simulink model "MBD2_problem3"  (R2020b)
settings: Solver=VariableStepAuto  StartTime=0.0  StopTime=100  RelTol=1e-3
InitFcn:
  | M = 1000;
  | b = 50;
  | u = 500;
  | Kp=1750;
  | Ki=800;
  | Ts=0.01;
settings Model: Creator=Lenovo  LastModifiedBy=Lenovo

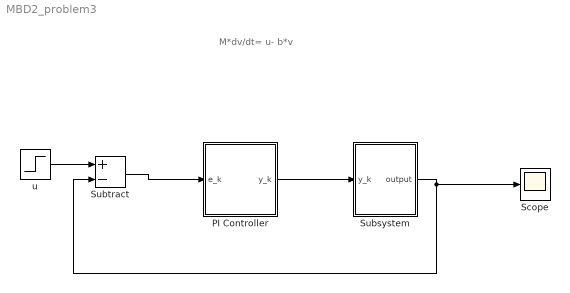
== system MBD2_problem3 ==
  note: M*dv/dt= u- b*v
  PI Controller : Subsystem
  Scope : Scope
  Subsystem : Subsystem
  Subtract : Sum  Inputs=+-
  u : Step  Time=0  SampleTime=0
  wires:
  Subsystem/1(output) -> Subtract/2, Scope/1
  u/1 -> Subtract/1
  Subtract/1 -> PI Controller/1(e_k)
  PI Controller/1(y_k) -> Subsystem/1(y_k)

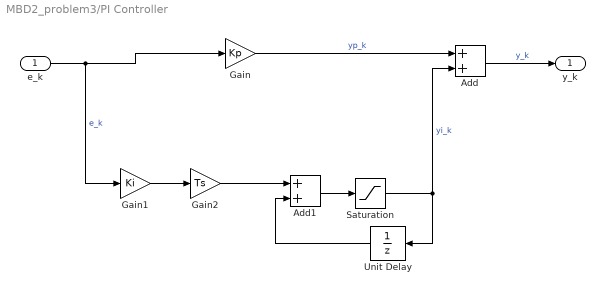
== system MBD2_problem3/PI Controller ==
  e_k : Inport  OutDataTypeStr=double  PortDimensions=1  SampleTime=0
  Add : Sum
  Add1 : Sum
  Gain : Gain  Gain=Kp
  Gain1 : Gain  Gain=Ki
  Gain2 : Gain  Gain=Ts
  Saturation : Saturate  UpperLimit=1  LowerLimit=-1
  Unit Delay : UnitDelay  SampleTime=-1  HasFrameUpgradeWarning=on
  y_k : Outport  OutDataTypeStr=double  PortDimensions=1  SampleTime=0
  wires:
  Gain2/1 -> Add1/1
  Add1/1 -> Saturation/1
  e_k/1 -> Gain/1, Gain1/1  "e_k"
  Gain1/1 -> Gain2/1
  Add/1 -> y_k/1  "y_k"
  Saturation/1 -> Unit Delay/1, Add/2  "yi_k"
  Gain/1 -> Add/1  "yp_k"
  Unit Delay/1 -> Add1/2

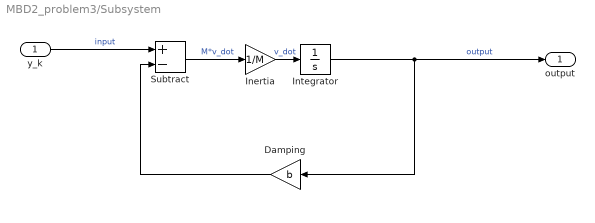
== system MBD2_problem3/Subsystem ==
  y_k : Inport
  Damping : Gain  Gain=b
  Inertia : Gain  Gain=1/M
  Integrator : Integrator
  Subtract : Sum  Inputs=+-
  output : Outport
  wires:
  Inertia/1 -> Integrator/1  "v_dot"
  Integrator/1 -> output/1, Damping/1  "output"
  Damping/1 -> Subtract/2
  Subtract/1 -> Inertia/1  "M*v_dot"
  y_k/1 -> Subtract/1  "input"
